simulink model "AC_base_1_VSM_2_22a"  (R2022a)
settings: Solver=ode3  StartTime=0.0  StopTime=8  FixedStep=HWSampleTime  RelTol=1e-3
undefined symbols (not defined in the file): ControlSampleTime, DiscIntNeverNeededParam, HWSampleTime, Ipwm_back, Ipwm_off, LCL, Manage, Oversample, Param, scaling_factor, SM, Ts, V_DC, VSMCTRL
libraries: fl_lib x100, nesl_utility x63, simulink x38, FriedrichLibrary x38, ee_lib x20, simulink_extras x14, TriphaseHardwaremodule x12, spsEdgeDetectorLib x2, StateMachines x2, slpidlib x2, spsPower3phInstantaneousLib x1
(part 6 of 7)

== system AC_base_1_VSM_2_22a/Variant Subsystem1/VSM/VSM1/VSM/MANAGEMENT/sp_VSM/PQ(U) Limit ==
  note: hier muss mit der Leistungsvorgabe multipliziert werden
      | 0.8 U * P0
  sp_PQ : Inport
  enable : Inport  Port=2
  u_out : Inport  Port=3
  Add : Sum
  Constant : Constant
  Dead Zone : DeadZone  LowerValue=0.95  UpperValue=1.05
  Demux : Demux  Outputs=2
  Demux1 : Demux  Outputs=2
  Math Function : Math  Operator=hypot  SignedPower=on
  MinMax : MinMax  Inputs=2
  Mux : Mux  Inputs=2
  Product : Product
  Scope : Scope
  Selector2 : Selector  InputPortWidth=3  IndexOptions=Index vector (dialog)  Indices=[1 2]  OutputSizes=1
  Switch : Switch  Criteria=u2 ~= 0  SaturateOnIntegerOverflow=off  InputSameDT=off
  sp_PQ_limit : Outport  VectorParamsAs1DForOutWhenUnconnected=off
  wires:
  Constant/1 -> Add/1
  Add/1 -> Product/1
  Dead Zone/1 -> Add/2
  Product/1 -> MinMax/1
  enable/1 -> Switch/2
  Switch/1 -> sp_PQ_limit/1, Scope/1
  Mux/1 -> Switch/1
  MinMax/1 -> Mux/1
  Demux1/1 -> Product/2, MinMax/2
  Demux1/2 -> Mux/2
  sp_PQ/1 -> Demux1/1, Switch/3
  u_out/1 -> Selector2/1
  Math Function/1 -> Dead Zone/1
  Demux/2 -> Math Function/2
  Demux/1 -> Math Function/1
  Selector2/1 -> Demux/1

== system AC_base_1_VSM_2_22a/Variant Subsystem1/VSM/VSM1/VSM/MANAGEMENT/sp_VSM/RateLimit ==
  PQ : Inport
  Enable : EnablePort
  Compare To Zero : simulink/Logic and Bit Operations/Compare To Zero  relop=>  OutDataTypeStr=boolean
  Constant1 : Constant  Value=Mgn.PQSpRateUp  SampleTime=ControlSampleTime
  Constant2 : Constant  Value=Mgn.PQSpRateDown  SampleTime=ControlSampleTime
  Constant6 : Constant  Value=Mgn.PQSpRateDown  SampleTime=ControlSampleTime
  Constant7 : Constant  Value=Mgn.PQSpRateUp  SampleTime=ControlSampleTime
  Constant8 : Constant  Value=[0 0]  SampleTime=ControlSampleTime
  Logical Operator : Logic  Inputs=1  AllPortsSameDT=off  OutDataTypeStr=boolean
  Mux : Mux  Inputs=2
  Switch : Switch  Criteria=u2 > Threshold  SaturateOnIntegerOverflow=off  InputSameDT=off
  ratelimitspPQ : Subsystem  mask{Ts=ControlSampleTime}
      mask DialogControl ParameterGroupVar Prompt: Rate Limiter
  PQslow : Outport  VectorParamsAs1DForOutWhenUnconnected=off
  wires:
  PQ/1 -> Switch/3, Switch/1, ratelimitspPQ/2(x)
  Constant8/1 -> ratelimitspPQ/4(x0)
  Constant6/1 -> ratelimitspPQ/3(ratedown)
  Switch/1 -> PQslow/1  "sp_PQ"
  Constant7/1 -> ratelimitspPQ/1(rateup)
  Compare To Zero/1 -> Logical Operator/1
  Constant1/1 -> Mux/1
  Constant2/1 -> Mux/2
  Mux/1 -> Compare To Zero/1
  Logical Operator/1 -> Switch/2

== system AC_base_1_VSM_2_22a/Variant Subsystem3/VSM/Inverter AverageMdl LC SimScape2/Modul F30 fixed DC voltage Average SimScape/simscape_bridgefilter_aca/PWM Blocking1/Trigger Spike at new Control Sample ==
  Add : Sum  Inputs=+-
  Compare To Constant : simulink/Logic and Bit Operations/Compare To Constant  relop=~=  const=0  OutDataTypeStr=boolean
  Rate Transition : RateTransition  OutPortSampleTime=ControlSampleTime
  Rate Transition1 : RateTransition  OutPortSampleTime=ControlSampleTime
  Rate Transition2 : RateTransition  OutPortSampleTime=ControlSampleTime/Oversample
  S-R Flip-Flop1 : simulink_extras/Flip Flops/S-R Flip-Flop  initial_condition=1
  Unit Delay : UnitDelay  SampleTime=-1  HasFrameUpgradeWarning=on
  Unit Delay2 : UnitDelay  SampleTime=-1  HasFrameUpgradeWarning=on
  Unit Delay3 : UnitDelay  SampleTime=-1  HasFrameUpgradeWarning=on
  y : Outport
  wires:
  S-R Flip-Flop1/1 -> Rate Transition2/1, Rate Transition/1
  Rate Transition2/1 -> Add/2, Unit Delay3/1
  S-R Flip-Flop1/2 -> Rate Transition1/1
  Unit Delay2/1 -> S-R Flip-Flop1/1
  Unit Delay3/1 -> Add/1
  Compare To Constant/1 -> y/1
  Add/1 -> Compare To Constant/1
  Unit Delay/1 -> S-R Flip-Flop1/2
  Rate Transition/1 -> Unit Delay/1
  Rate Transition1/1 -> Unit Delay2/1

== system AC_base_1_VSM_2_22a/Variant Subsystem3/VSM/Inverter AverageMdl LC SimScape2/Modul F30 fixed DC voltage Average SimScape/simscape_bridgefilter_aca1/PWM Blocking1/Trigger Spike at new Control Sample ==
  Add : Sum  Inputs=+-
  Compare To Constant : simulink/Logic and Bit Operations/Compare To Constant  relop=~=  const=0  OutDataTypeStr=boolean
  Rate Transition : RateTransition  OutPortSampleTime=ControlSampleTime
  Rate Transition1 : RateTransition  OutPortSampleTime=ControlSampleTime
  Rate Transition2 : RateTransition  OutPortSampleTime=ControlSampleTime/Oversample
  S-R Flip-Flop1 : simulink_extras/Flip Flops/S-R Flip-Flop  initial_condition=1
  Unit Delay : UnitDelay  SampleTime=-1  HasFrameUpgradeWarning=on
  Unit Delay2 : UnitDelay  SampleTime=-1  HasFrameUpgradeWarning=on
  Unit Delay3 : UnitDelay  SampleTime=-1  HasFrameUpgradeWarning=on
  y : Outport
  wires:
  Rate Transition1/1 -> Unit Delay2/1
  Rate Transition/1 -> Unit Delay/1
  Unit Delay/1 -> S-R Flip-Flop1/2
  Add/1 -> Compare To Constant/1
  Compare To Constant/1 -> y/1
  Unit Delay3/1 -> Add/1
  Unit Delay2/1 -> S-R Flip-Flop1/1
  S-R Flip-Flop1/2 -> Rate Transition1/1
  Rate Transition2/1 -> Unit Delay3/1, Add/2
  S-R Flip-Flop1/1 -> Rate Transition/1, Rate Transition2/1

== system AC_base_1_VSM_2_22a/Variant Subsystem3/VSM/Inverter AverageMdl LC SimScape2/Modul F30 fixed DC voltage Average SimScape/simscape_bridgefilter_aca2/PWM Blocking1/Trigger Spike at new Control Sample ==
  Add : Sum  Inputs=+-
  Compare To Constant : simulink/Logic and Bit Operations/Compare To Constant  relop=~=  const=0  OutDataTypeStr=boolean
  Rate Transition : RateTransition  OutPortSampleTime=ControlSampleTime
  Rate Transition1 : RateTransition  OutPortSampleTime=ControlSampleTime
  Rate Transition2 : RateTransition  OutPortSampleTime=ControlSampleTime/Oversample
  S-R Flip-Flop1 : simulink_extras/Flip Flops/S-R Flip-Flop  initial_condition=1
  Unit Delay : UnitDelay  SampleTime=-1  HasFrameUpgradeWarning=on
  Unit Delay2 : UnitDelay  SampleTime=-1  HasFrameUpgradeWarning=on
  Unit Delay3 : UnitDelay  SampleTime=-1  HasFrameUpgradeWarning=on
  y : Outport
  wires:
  S-R Flip-Flop1/1 -> Rate Transition2/1, Rate Transition/1
  Rate Transition2/1 -> Add/2, Unit Delay3/1
  S-R Flip-Flop1/2 -> Rate Transition1/1
  Unit Delay2/1 -> S-R Flip-Flop1/1
  Unit Delay3/1 -> Add/1
  Compare To Constant/1 -> y/1
  Add/1 -> Compare To Constant/1
  Unit Delay/1 -> S-R Flip-Flop1/2
  Rate Transition/1 -> Unit Delay/1
  Rate Transition1/1 -> Unit Delay2/1

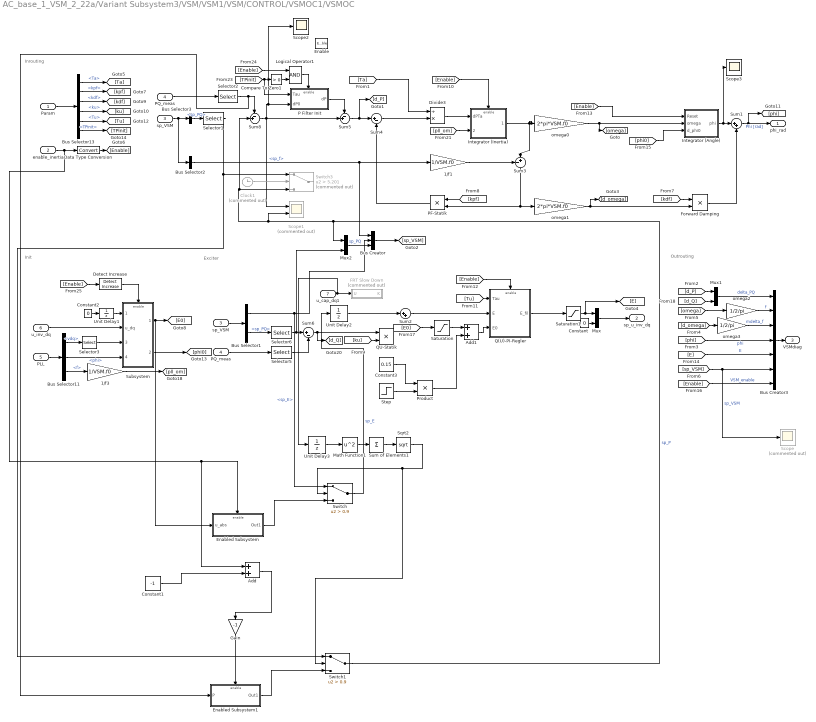
== system AC_base_1_VSM_2_22a/Variant Subsystem3/VSM/VSM1/VSM/CONTROL/VSMOC1/VSMOC ==
  note: Inrouting
  note: Exciter
  note: Init
  note: Outrouting
  Param : Inport
  enable_inertia : Inport  Port=2
  sp_VSM : Inport  Port=3
  PQ_meas : Inport  Port=4
  PLL : Inport  Port=5
  u_inv_dq : Inport  Port=6
  u_cap_dq1 : Inport  Port=7
  Enable : EnablePort  StatesWhenEnabling=reset
  1/f1 : Gain  Gain=1/VSM.f0
  1/f3 : Gain  Gain=1/VSM.f0
  Add : Sum
  Add1 : Sum
  Bus Creator : BusCreator  Inputs=3
  Bus Creator3 : BusCreator  Inputs=7
  Bus Selector1 : BusSelector  OutputSignals=sp_E,sp_PQ
  Bus Selector11 : BusSelector  OutputSignals=vdq,phi,f
  Bus Selector13 : BusSelector  OutputSignals=Ta,kpf,kdf,ku,Tu,TPinit
  Bus Selector2 : BusSelector  OutputSignals=sp_f
  Bus Selector3 : BusSelector  OutputSignals=sp_PQ
  Clock1 : Clock  Commented=on
  Compare To Zero1 : simulink/Logic and Bit Operations/Compare To Zero  relop=>  OutDataTypeStr=boolean
  Constant : Constant  Value=0
  Constant1 : Constant  Value=-1
  Constant2 : Constant  Value=0  SampleTime=ControlSampleTime
  Constant3 : Constant  Value=0.15
  Data Type Conversion : DataTypeConversion  SaturateOnIntegerOverflow=off  RndMeth=Floor
  Detect Increase : simulink/Logic and Bit Operations/Detect Increase  vinit=0.0  OutDataTypeStr=boolean
  Divide3 : Product  Inputs=/*
  Enabled Subsystem : Subsystem  TreatAsAtomicUnit=on
  Enabled Subsystem1 : Subsystem  TreatAsAtomicUnit=on
  FRT Slow Down : Subsystem  Commented=on
  Forward Damping : Product  Inputs=**
  Gain : Gain  Gain=-1
  Integrator (Angle) : Subsystem
  Integrator (Inertia) : Subsystem
  Logical Operator1 : Logic  AllPortsSameDT=off  OutDataTypeStr=boolean
  Math Function1 : Math  Operator=square  SignedPower=on
  Mux : Mux  Inputs=2
  Mux1 : Mux  Inputs=2
  Mux2 : Mux  Inputs=2
  P Filter Init : Subsystem
  PF-Statik : Product  Inputs=**
  "PQ_meas " : InportShadow  Port=4
  Product : Product
  Q(U)-PI-Regler : Subsystem
  QU-Statik : Product  Inputs=**
  Saturation : Saturate  UpperLimit=1.8  LowerLimit=0.8*0
  Saturation1 : Saturate  UpperLimit=2
  Scope : Scope  Commented=on
  Scope1 : Scope  Commented=on  NumInputPorts=2
  Scope2 : Scope
  Scope3 : Scope
  Selector1 : Selector  InputPortWidth=2  IndexOptions=Index vector (dialog)  Indices=1  OutputSizes=1
  Selector2 : Selector  InputPortWidth=2  IndexOptions=Index vector (dialog)  Indices=1  OutputSizes=1
  Selector3 : Selector  InputPortWidth=3  IndexOptions=Index vector (dialog)  Indices=[1 2]  OutputSizes=1
  Selector5 : Selector  InputPortWidth=2  IndexOptions=Index vector (dialog)  Indices=2  OutputSizes=1
  Selector6 : Selector  InputPortWidth=2  IndexOptions=Index vector (dialog)  Indices=2  OutputSizes=1
  Sqrt2 : Sqrt
  Step : Step  Time=2  After=0  SampleTime=0
  Subsystem : Subsystem
  Sum of Elements1 : Sum  Inputs=+
  Sum1 : Sum  Inputs=|++
  Sum2 : Sum  Inputs=|++
  Sum3 : Sum  Inputs=-+|
  Sum4 : Sum  Inputs=|+-
  Sum5 : Sum  Inputs=-+|
  Sum6 : Sum  Inputs=|+-
  Sum8 : Sum  Inputs=-+|
  Switch : Switch  Criteria=u2 > Threshold  Threshold=0.9  SaturateOnIntegerOverflow=off  InputSameDT=off
  Switch1 : Switch  Criteria=u2 > Threshold  Threshold=0.9  SaturateOnIntegerOverflow=off  InputSameDT=off
  Switch3 : Switch  Commented=on  Criteria=u2 > Threshold  Threshold=5.201  SaturateOnIntegerOverflow=off  InputSameDT=off
  Unit Delay1 : UnitDelay  InitialCondition=1  SampleTime=ControlSampleTime  HasFrameUpgradeWarning=on
  Unit Delay2 : UnitDelay  SampleTime=-1  HasFrameUpgradeWarning=on
  Unit Delay3 : UnitDelay  SampleTime=-1  HasFrameUpgradeWarning=on
  omega0 : Gain  Gain=2*pi*VSM.f0
  omega1 : Gain  Gain=2*pi*VSM.f0
  omega2 : Gain  Gain=1/2/pi
  omega3 : Gain  Gain=1/2/pi
  "sp_VSM " : InportShadow  Port=3
  phi_rad : Outport  VectorParamsAs1DForOutWhenUnconnected=off
  sp_u_inv_dq : Outport  Port=2  InitialOutput=[1 0]  VectorParamsAs1DForOutWhenUnconnected=off
  VSMdiag : Outport  Port=3  VectorParamsAs1DForOutWhenUnconnected=off
  wires:
  [Enable] -> Q(U)-PI-Regler/Enable
  Bus Selector11/2 -> Subsystem/4(phi_pll)  "<phi>"
  Selector5/1 -> Sum6/2
  Selector6/1 -> Mux2/2, Sum6/1
  1/f1/1 -> Sum3/1
  [d_Q] -> Mux1/2
  [d_P] -> Mux1/1
  Mux1/1 -> Bus Creator3/1  "delta_PQ"
  Selector2/1 -> Enabled Subsystem1/1(P), Sum8/1
  Sum6/1 -> QU-Statik/1, [d_Q]
  "sp_VSM "/1 -> Bus Selector1/1
  Bus Selector1/2 -> Selector6/1  "<sp_PQ>"
  "PQ_meas "/1 -> Selector5/1
  [kpf] -> PF-Statik/1
  [kdf] -> Forward Damping/1
  1/f3/1 -> [pll_om]
  Bus Selector11/3 -> 1/f3/1  "<f>"
  Integrator (Angle)/1(phi) -> Scope3/1, Sum1/1
  Selector3/1 -> Subsystem/3(u_dq_pll)
  [Enable] -> Bus Creator3/7  "VSM_enable"
  Sum1/1 -> [phi], phi_rad/1  "Phi [rad]"
  Sum4/1 -> Divide3/2
  Sum3/1 -> PF-Statik/2, omega1/1
  Bus Selector2/1 -> Bus Creator/1, 1/f1/1  "<sp_f>"
  PLL/1 -> Bus Selector11/1
  Bus Creator3/1 -> VSMdiag/1
  [omega] -> omega2/1
  omega1/1 -> Forward Damping/2, [d_omega]
  [d_omega] -> omega3/1
  omega2/1 -> Bus Creator3/2  "f"
  omega3/1 -> Bus Creator3/3  "mdelta_f"
  [sp_VSM] -> Scope/1, Bus Creator3/6  "sp_VSM"
  PQ_meas/1 -> Selector2/1
  Bus Selector11/1 -> Selector3/1  "<vdq>"
  Divide3/1 -> Integrator (Inertia)/1(dPTa)
  [pll_om] -> Integrator (Inertia)/2(omega0 [pu])
  Mux/1 -> sp_u_inv_dq/1
  Constant/1 -> Mux/2
  Subsystem/2(u_ang) -> [phi0]
  Detect Increase/1 -> Subsystem/Enable
  Sum5/1 -> Sum4/1, [d_P]
  [TPinit] -> P Filter Init/1(Tau), Compare To Zero1/1
  Compare To Zero1/1 -> Logical Operator1/2
  Logical Operator1/1 -> P Filter Init/Enable
  [Enable] -> Logical Operator1/1
  Bus Selector13/5 -> [Tu]  "<Tu>"
  Bus Selector13/4 -> [ku]  "<ku>"
  Bus Selector13/3 -> [kdf]  "<kdf>"
  Bus Selector13/2 -> [kpf]  "<kpf>"
  Bus Selector13/1 -> [Ta]  "<Ta>"
  Param/1 -> Bus Selector13/1
  [Enable] -> Detect Increase/1
  u_inv_dq/1 -> Subsystem/2(u_dq)
  Constant2/1 -> Unit Delay1/1
  Unit Delay1/1 -> Subsystem/1(first_run)
  Data Type Conversion/1 -> [Enable]
  Sum2/1 -> Q(U)-PI-Regler/2(E)
  [ku] -> QU-Statik/2
  [E] -> Bus Creator3/5  "E"
  Bus Selector13/6 -> [TPinit]  "<TPinit>"
  [phi] -> Bus Creator3/4  "phi"
  [Tu] -> Q(U)-PI-Regler/1(Tau)
  Unit Delay2/1 -> Sum2/1
  [E0] -> Saturation/1
  [Enable] -> Integrator (Angle)/1(Reset)
  omega0/1 -> Integrator (Angle)/2(omega), [omega]
  Saturation1/1 -> [E], Mux/1
  Forward Damping/1 -> Sum1/2
  [Enable] -> Integrator (Inertia)/Enable
  Integrator (Inertia)/1(omega [pu]) -> omega0/1, Sum3/2
  Bus Selector3/1 -> Selector1/1  "<sp_PQ>"
  sp_VSM/1 -> Bus Selector2/1, Bus Selector3/1
  Sum8/1 -> Scope1/1, Sum5/2, Scope2/1, P Filter Init/2(dP0)
  [phi0] -> Integrator (Angle)/3(d_phi0)
  [Ta] -> Divide3/1
  P Filter Init/1(dP) -> Sum5/1
  PF-Statik/1 -> Sum4/2
  Sqrt2/1 -> Switch1/2, Switch/2
  u_cap_dq1/1 -> Unit Delay3/1, FRT Slow Down/1(U)
  Sum of Elements1/1 -> Sqrt2/1
  Unit Delay3/1 -> Math Function1/1
  Math Function1/1 -> Sum of Elements1/1
  Bus Selector1/1 -> Bus Creator/2, Switch/1  "<sp_E>"
  enable_inertia/1 -> Add/1, Enabled Subsystem/Enable, Data Type Conversion/1
  Enabled Subsystem/1(Out1) -> Switch/3
  Subsystem/1(u_abs) -> Enabled Subsystem/1(u_abs), [E0]
  Enabled Subsystem1/1(Out1) -> Switch1/3
  Switch/1 -> Unit Delay2/1  "sp_E"
  Switch1/1 -> Scope1/2, Sum8/2, Switch3/3, Mux2/1  "sp_P"
  Clock1/1 -> Switch3/2
  Q(U)-PI-Regler/1(E_fil) -> Saturation1/1
  Selector1/1 -> Switch3/1, Switch1/1
  Constant1/1 -> Add/2
  Gain/1 -> Enabled Subsystem1/Enable
  Add/1 -> Gain/1
  Saturation/1 -> Add1/1
  Add1/1 -> Q(U)-PI-Regler/3(E0)
  Step/1 -> Product/2
  Constant3/1 -> Product/1
  Product/1 -> Add1/2
  Mux2/1 -> Bus Creator/3  "sp_PQ"
  Bus Creator/1 -> [sp_VSM]

== system AC_base_1_VSM_2_22a/Variant Subsystem3/VSM/VSM1/VSM/CONTROL/Virtual Circuit mit R und L/Current Predictor ==
  u : Inport
  Delay : Delay  DelayLength=1  InitialCondition=0
  Sum : Sum  Inputs=|-+
  Sum1 : Sum  Inputs=|++
  y : Outport
  wires:
  u/1 -> Sum/2, Sum1/2, Delay/1
  Delay/1 -> Sum/1
  Sum/1 -> Sum1/1
  Sum1/1 -> y/1

== system AC_base_1_VSM_2_22a/Variant Subsystem3/VSM/VSM1/VSM/CONTROL/Virtual Circuit mit R und L/PT1 ==
  U : Inport  SampleTime=Ts
  tau : Inport  Port=2  SampleTime=Ts
  Reset : Inport  Port=3  SampleTime=Ts
  Phi : Inport  Port=4
  Delay : Delay  DelayLength=1  InitialConditionSource=Input port  ExternalReset=Rising
      settings: InputPortMap=u0,r5,p4
  Divide : Product  Inputs=*/
  Gain : Gain  Gain=Ts
  Gain1 : Gain  Gain=K
  Saturation : Saturate  UpperLimit=inf  LowerLimit=Ts
  Sum : Sum  Inputs=|++
  Sum2 : Sum  Inputs=|+-
  Unit Delay2 : UnitDelay  InitialCondition=[0 0 0]  SampleTime=ControlSampleTime  HasFrameUpgradeWarning=on
  dq0->ab0 phi : FriedrichLibrary/Transformations/dq0->ab0 phi  SystemSampleTime=-1  VariantActivationTime=update diagram  Latency=0  AutoFrameSizeCalculation=off
  Y : Outport
  wires:
  Phi/1 -> dq0->ab0 phi/2
  Unit Delay2/1 -> dq0->ab0 phi/1
  Sum/1 -> Gain1/1, Unit Delay2/1, Delay/1
  Reset/1 -> Delay/2
  Saturation/1 -> Divide/2
  Divide/1 -> Sum/1
  tau/1 -> Saturation/1
  Delay/1 -> Sum2/2, Sum/2
  Gain/1 -> Divide/1
  U/1 -> Sum2/1
  Sum2/1 -> Gain/1
  Gain1/1 -> Y/1
  dq0->ab0 phi/1 -> Delay/3

== system AC_base_1_VSM_2_22a/Variant Subsystem3/VSM/VSM1/VSM/CONTROL/Virtual Circuit mit R und L/PT2 ==
  U : Inport  SampleTime=Ts
  tau : Inport  Port=2  SampleTime=Ts
  Reset : Inport  Port=3  SampleTime=Ts
  Phi : Inport  Port=4
  Delay : Delay  DelayLength=1  InitialConditionSource=Input port  ExternalReset=Rising
      settings: InputPortMap=u0,r5,p4
  Divide : Product  Inputs=*/
  Gain : Gain  Gain=Ts
  Gain1 : Gain  Gain=K
  Saturation : Saturate  UpperLimit=inf  LowerLimit=Ts
  Sum : Sum  Inputs=|++
  Sum2 : Sum  Inputs=|+-
  Unit Delay2 : UnitDelay  InitialCondition=[0 0 0]  SampleTime=ControlSampleTime  HasFrameUpgradeWarning=on
  dq0->ab0 phi1 : FriedrichLibrary/Transformations/dq0->ab0 phi  SystemSampleTime=-1  VariantActivationTime=update diagram  Latency=0  AutoFrameSizeCalculation=off
  Y : Outport
  wires:
  dq0->ab0 phi1/1 -> Delay/3
  Gain1/1 -> Y/1
  Sum2/1 -> Gain/1
  U/1 -> Sum2/1
  Gain/1 -> Divide/1
  Delay/1 -> Sum/2, Sum2/2
  tau/1 -> Saturation/1
  Divide/1 -> Sum/1
  Saturation/1 -> Divide/2
  Reset/1 -> Delay/2
  Sum/1 -> Delay/1, Unit Delay2/1, Gain1/1
  Unit Delay2/1 -> dq0->ab0 phi1/1
  Phi/1 -> dq0->ab0 phi1/2

== system AC_base_1_VSM_2_22a/Variant Subsystem3/VSM/VSM1/VSM/CONTROL/Virtual Circuit1/Current Predictor ==
  u : Inport
  Delay : Delay  DelayLength=1  InitialCondition=0
  Sum : Sum  Inputs=|-+
  Sum1 : Sum  Inputs=|++
  y : Outport
  wires:
  u/1 -> Sum/2, Sum1/2, Delay/1
  Delay/1 -> Sum/1
  Sum/1 -> Sum1/1
  Sum1/1 -> y/1

== system AC_base_1_VSM_2_22a/Variant Subsystem3/VSM/VSM1/VSM/CONTROL/Virtual Circuit1/PT1 ==
  U : Inport  SampleTime=Ts
  tau : Inport  Port=2  SampleTime=Ts
  Reset : Inport  Port=3  SampleTime=Ts
  Delay : Delay  DelayLength=1
  Divide : Product  Inputs=*/
  Gain : Gain  Gain=Ts
  Gain1 : Gain  Gain=K
  Saturation : Saturate  UpperLimit=inf  LowerLimit=Ts
  Sum : Sum  Inputs=|++
  Sum2 : Sum  Inputs=|+-
  Switch : Switch  Criteria=u2 > Threshold  SaturateOnIntegerOverflow=off  InputSameDT=off
  Y : Outport
  wires:
  Reset/1 -> Switch/2
  Saturation/1 -> Divide/2
  Divide/1 -> Sum/1
  tau/1 -> Saturation/1
  Delay/1 -> Sum2/2, Sum/2
  Gain/1 -> Divide/1
  U/1 -> Switch/1, Sum2/1
  Sum2/1 -> Gain/1
  Gain1/1 -> Y/1
  Switch/1 -> Gain1/1, Delay/1
  Sum/1 -> Switch/3

== system AC_base_1_VSM_2_22a/Variant Subsystem3/VSM/VSM1/VSM/CONTROL/Virtual Circuit1/PT2 ==
  U : Inport  SampleTime=Ts
  tau : Inport  Port=2  SampleTime=Ts
  Reset : Inport  Port=3  SampleTime=Ts
  Phi : Inport  Port=4
  Delay : Delay  DelayLength=1  InitialConditionSource=Input port  ExternalReset=Rising
      settings: InputPortMap=u0,r5,p4
  Divide : Product  Inputs=*/
  Gain : Gain  Gain=Ts
  Gain1 : Gain  Gain=K
  Saturation : Saturate  UpperLimit=inf  LowerLimit=Ts
  Sum : Sum  Inputs=|++
  Sum2 : Sum  Inputs=|+-
  Unit Delay2 : UnitDelay  InitialCondition=[0 0 0]  SampleTime=ControlSampleTime  HasFrameUpgradeWarning=on
  dq0->ab0 phi1 : FriedrichLibrary/Transformations/dq0->ab0 phi  SystemSampleTime=-1  VariantActivationTime=update diagram  Latency=0  AutoFrameSizeCalculation=off
  Y : Outport
  wires:
  dq0->ab0 phi1/1 -> Delay/3
  Gain1/1 -> Y/1
  Sum2/1 -> Gain/1
  U/1 -> Sum2/1
  Gain/1 -> Divide/1
  Delay/1 -> Sum/2, Sum2/2
  tau/1 -> Saturation/1
  Divide/1 -> Sum/1
  Saturation/1 -> Divide/2
  Reset/1 -> Delay/2
  Sum/1 -> Delay/1, Unit Delay2/1, Gain1/1
  Unit Delay2/1 -> dq0->ab0 phi1/1
  Phi/1 -> dq0->ab0 phi1/2

== system AC_base_1_VSM_2_22a/Variant Subsystem3/VSM/VSM1/VSM/CONTROL/i_dq_ctrl/PI ==
  di : Inport
  u0 : Inport  Port=2
  Enable : EnablePort  StatesWhenEnabling=reset
  Gain4 : Gain  Gain=Ki
  Gain5 : Gain  Gain=Kp
  Integrator (inertia) : DiscreteIntegrator  gainval=1  InitialConditionSource=external  InitialCondition=1  SampleTime=ControlSampleTime  ICPrevOutput=DiscIntNeverNeededParam  ICPrevScaledInput=DiscIntNeverNeededParam
  Product : Product
  Product1 : Product
  Step : Step  Time=8  Before=1  SampleTime=0
  Step1 : Step  Time=8.05+10  Before=1  After=0.1  SampleTime=0
  Sum2 : Sum  Inputs=++|
  u : Outport  VectorParamsAs1DForOutWhenUnconnected=off
  wires:
  u0/1 -> Integrator (inertia)/2
  Sum2/1 -> u/1
  di/1 -> Gain4/1, Gain5/1
  Integrator (inertia)/1 -> Sum2/2
  Gain5/1 -> Product/2
  Gain4/1 -> Product1/2
  Product1/1 -> Integrator (inertia)/1
  Product/1 -> Sum2/1
  Step/1 -> Product/1
  Step1/1 -> Product1/1

== system AC_base_1_VSM_2_22a/Variant Subsystem3/VSM/VSM1/VSM/MANAGEMENT/Subsystem1/Enabled Subsystem ==
  i_abs : Inport
  i_pq : Inport  Port=2
  Enable : EnablePort
  i abs_pre : Outport
  i_pq_pre : Outport  Port=2
  wires:
  i_abs/1 -> i abs_pre/1
  i_pq/1 -> i_pq_pre/1

== system AC_base_1_VSM_2_22a/Variant Subsystem3/VSM/VSM1/VSM/MANAGEMENT/Subsystem1/Subsystem ==
  note: für mean muss simscape installiert sein
  note: zweiter Faktor bei clearing für richtiges Q
      |
      | bei Eintritt mit Halten aber fester Grenze
      |
      | bis jetzt über Zeit abgeschaltet bei clearing ohne Halten
  i_inv : Inport
  PQ_out : Inport  Port=2
  iabs : Inport  Port=3
  U_cap : Inport  Port=4
  PQ_pre : Inport  Port=5
  i abs_pre : Inport  Port=6
  angle_i : Inport  Port=7
  Enable : EnablePort
  Abs : Abs  SaturateOnIntegerOverflow=off
  Add : Sum  Inputs=+-
  Clock : Clock
  Complex to Magnitude-Angle : ComplexToMagnitudeAngle
  Demux1 : Demux  Outputs=2
  Discrete Derivative2 : simulink/Discrete/Discrete Derivative  gainval=1.0  ICPrevScaledInput=0.0  OutMin=[]  OutMax=[]  OutDataType=fixdt(1, 16)  OutScaling=2^-10  DoSatur=off
  Discrete-Time Integrator : DiscreteIntegrator  SampleTime=-1  ICPrevOutput=DiscIntNeverNeededParam  ICPrevScaledInput=DiscIntNeverNeededParam
  Divide2 : Product  Inputs=*/
  Gain : Gain  Gain=1000  SaturateOnIntegerOverflow=on  OutDataTypeStr=Inherit: Same as input  ParamDataTypeStr=Inherit: Same as input
  K1 : Constant  Value=1./1000  SampleTime=Ts
  MATLAB Function1 : MATLAB Function  TreatAsAtomicUnit=on  SystemSampleTime=ControlSampleTime
  MATLAB Function2 : MATLAB Function  Commented=on  TreatAsAtomicUnit=on  SystemSampleTime=ControlSampleTime
  Memory : Memory
  Real-Imag to Complex : RealImagToComplex
  Relational Operator : RelationalOperator  OutDataTypeStr=boolean  ZeroCross=off  SampleTime=Ts  InputSameDT=off
  Scope1 : Scope  NumInputPorts=2
  Scope2 : Scope  NumInputPorts=2
  Selector3 : Selector  InputPortWidth=2  IndexOptions=Index vector (dialog)  Indices=2  OutputSizes=1
  Signal Specification9 : SignalSpecification  Dimensions=[1 2]
  Sum : Sum  Inputs=+-  InputSameDT=on  SaturateOnIntegerOverflow=on  OutDataTypeStr=Inherit: Same as first input
  Switch : Switch  Threshold=0.5  SaturateOnIntegerOverflow=off
  Transport Delay : TransportDelay  DelayTime=0.002
  Transport Delay1 : TransportDelay  DelayTime=1./1000  BufferSize=2048*4  PadeOrder=2
  i_sp : Outport
  CC : Outport  Port=2
  set : Outport  Port=3
  wires:
  PQ_out/1 -> MATLAB Function1/2(PQ_out), Divide2/1
  iabs/1 -> MATLAB Function1/3(i_abs)
  U_cap/1 -> MATLAB Function1/5(U_cap), Divide2/2, Add/1, Transport Delay/1
  MATLAB Function1/1(i_sp) -> Signal Specification9/1
  MATLAB Function1/2(CC) -> CC/1
  i abs_pre/1 -> MATLAB Function1/7(i_abs_pre)
  Transport Delay/1 -> Add/2
  Add/1 -> MATLAB Function1/8(u_diff)
  i_inv/1 -> MATLAB Function1/1(i_inv)
  Discrete Derivative2/1 -> Abs/1
  MATLAB Function1/3(set1) -> set/1, Scope1/1
  Divide2/1 -> Selector3/1, Scope2/1
  Selector3/1 -> Discrete Derivative2/1
  Demux1/1 -> Real-Imag to Complex/1
  PQ_pre/1 -> MATLAB Function1/6(i_pq_pre), Demux1/1
  Complex to Magnitude-Angle/2 -> MATLAB Function1/9(angle_pre)
  Demux1/2 -> Real-Imag to Complex/2
  Real-Imag to Complex/1 -> Complex to Magnitude-Angle/1
  angle_i/1 -> MATLAB Function1/10(angle_i)
  Signal Specification9/1 -> i_sp/1
  Relational Operator/1 -> Switch/2
  Memory/1 -> Switch/3
  Discrete-Time Integrator/1 -> Sum/1, Transport Delay1/1
  Sum/1 -> Gain/1
  Gain/1 -> Switch/1
  Clock/1 -> Relational Operator/1
  K1/1 -> Relational Operator/2
  Transport Delay1/1 -> Sum/2
  Abs/1 -> Discrete-Time Integrator/1
  Switch/1 -> MATLAB Function1/4(der), Scope2/2, Memory/1

== system AC_base_1_VSM_2_22a/Variant Subsystem3/VSM/VSM1/VSM/MANAGEMENT/sp_VSM/E(PQ) ==
  E : Inport
  cmd : Inport  Port=2
  sp_PQ : Inport  Port=3
  Abs : Abs  SaturateOnIntegerOverflow=off
  Add : Sum
  Add1 : Sum  Inputs=--
  Add2 : Sum  Inputs=+++
  Bus Selector : BusSelector  OutputSignals=Param.VC.R1,Param.VC.R1t,Param.VC.L1,Param.VC.L1t,Param.VSM.ku
  Bus Selector1 : BusSelector  OutputSignals=Param.VSM.sp_E_comp
  Constant : Constant
  Demux : Demux  Outputs=2
  Display{,1..4} (5 alike) : Display
  Divide : Product  Inputs=/*
  Product : Product
  Product1 : Product
  Real-Imag to Complex : RealImagToComplex
  Real-Imag to Complex1 : RealImagToComplex
  Switch : Switch  Criteria=u2 ~= 0  SaturateOnIntegerOverflow=off  InputSameDT=off
  "cmd " : InportShadow  Port=2
  sp_E : Outport  VectorParamsAs1DForOutWhenUnconnected=off
  wires:
  Add2/1 -> Display3/1, Abs/1
  Abs/1 -> Display4/1, Switch/1
  Product/1 -> Display2/1, Add2/2  "voltage"
  Real-Imag to Complex/1 -> Display1/1, Product/2  "impedance"
  Divide/1 -> Display/1, Product/1  "current"
  Real-Imag to Complex1/1 -> Divide/2
  Demux/2 -> Product1/1, Real-Imag to Complex1/2
  Demux/1 -> Real-Imag to Complex1/1
  sp_PQ/1 -> Demux/1
  E/1 -> Switch/3
  Add1/1 -> Real-Imag to Complex/2
  Add/1 -> Real-Imag to Complex/1
  Bus Selector/4 -> Add1/2  "<L1t>"
  Bus Selector/3 -> Add1/1  "<L1>"
  Bus Selector/2 -> Add/2  "<R1t>"
  Bus Selector/1 -> Add/1  "<R1>"
  cmd/1 -> Bus Selector/1
  Switch/1 -> sp_E/1
  "cmd "/1 -> Bus Selector1/1
  Bus Selector1/1 -> Switch/2  "<sp_E_comp>"
  Bus Selector/5 -> Product1/2  "<ku>"
  Product1/1 -> Add2/3
  Constant/1 -> Divide/1, Add2/1

== system AC_base_1_VSM_2_22a/Variant Subsystem3/VSM/VSM1/VSM/MANAGEMENT/sp_VSM/PQ(U) Limit ==
  note: hier muss mit der Leistungsvorgabe multipliziert werden
      | 0.8 U * P0
  sp_PQ : Inport
  enable : Inport  Port=2
  u_out : Inport  Port=3
  Add : Sum
  Constant : Constant
  Dead Zone : DeadZone  LowerValue=0.95  UpperValue=1.05
  Demux : Demux  Outputs=2
  Demux1 : Demux  Outputs=2
  Math Function : Math  Operator=hypot  SignedPower=on
  MinMax : MinMax  Inputs=2
  Mux : Mux  Inputs=2
  Product : Product
  Scope : Scope
  Selector2 : Selector  InputPortWidth=3  IndexOptions=Index vector (dialog)  Indices=[1 2]  OutputSizes=1
  Switch : Switch  Criteria=u2 ~= 0  SaturateOnIntegerOverflow=off  InputSameDT=off
  sp_PQ_limit : Outport  VectorParamsAs1DForOutWhenUnconnected=off
  wires:
  Selector2/1 -> Demux/1
  Demux/1 -> Math Function/1
  Demux/2 -> Math Function/2
  Math Function/1 -> Dead Zone/1
  u_out/1 -> Selector2/1
  sp_PQ/1 -> Switch/3, Demux1/1
  Demux1/2 -> Mux/2
  Demux1/1 -> MinMax/2, Product/2
  MinMax/1 -> Mux/1
  Mux/1 -> Switch/1
  Switch/1 -> Scope/1, sp_PQ_limit/1
  enable/1 -> Switch/2
  Product/1 -> MinMax/1
  Dead Zone/1 -> Add/2
  Add/1 -> Product/1
  Constant/1 -> Add/1

== system AC_base_1_VSM_2_22a/Variant Subsystem3/VSM/VSM1/VSM/MANAGEMENT/sp_VSM/RateLimit ==
  PQ : Inport
  Enable : EnablePort
  Compare To Zero : simulink/Logic and Bit Operations/Compare To Zero  relop=>  OutDataTypeStr=boolean
  Constant1 : Constant  Value=Mgn.PQSpRateUp  SampleTime=ControlSampleTime
  Constant2 : Constant  Value=Mgn.PQSpRateDown  SampleTime=ControlSampleTime
  Constant6 : Constant  Value=Mgn.PQSpRateDown  SampleTime=ControlSampleTime
  Constant7 : Constant  Value=Mgn.PQSpRateUp  SampleTime=ControlSampleTime
  Constant8 : Constant  Value=[0 0]  SampleTime=ControlSampleTime
  Logical Operator : Logic  Inputs=1  AllPortsSameDT=off  OutDataTypeStr=boolean
  Mux : Mux  Inputs=2
  Switch : Switch  Criteria=u2 > Threshold  SaturateOnIntegerOverflow=off  InputSameDT=off
  ratelimitspPQ : Subsystem  mask{Ts=ControlSampleTime}
      mask DialogControl ParameterGroupVar Prompt: Rate Limiter
  PQslow : Outport  VectorParamsAs1DForOutWhenUnconnected=off
  wires:
  Logical Operator/1 -> Switch/2
  Mux/1 -> Compare To Zero/1
  Constant2/1 -> Mux/2
  Constant1/1 -> Mux/1
  Compare To Zero/1 -> Logical Operator/1
  Constant7/1 -> ratelimitspPQ/1(rateup)
  Switch/1 -> PQslow/1  "sp_PQ"
  Constant6/1 -> ratelimitspPQ/3(ratedown)
  Constant8/1 -> ratelimitspPQ/4(x0)
  PQ/1 -> ratelimitspPQ/2(x), Switch/1, Switch/3

== system AC_base_1_VSM_2_22a/Variant Subsystem1/VSM/VSM1/VSM/CONTROL/VSMOC1/VSMOC/Enabled Subsystem ==
  u_abs : Inport
  Enable : EnablePort
  Out1 : Outport
  wires:
  u_abs/1 -> Out1/1

== system AC_base_1_VSM_2_22a/Variant Subsystem1/VSM/VSM1/VSM/CONTROL/VSMOC1/VSMOC/Enabled Subsystem1 ==
  P : Inport
  Enable : EnablePort
  Out1 : Outport
  wires:
  P/1 -> Out1/1

== system AC_base_1_VSM_2_22a/Variant Subsystem1/VSM/VSM1/VSM/CONTROL/VSMOC1/VSMOC/FRT Slow Down ==
  U : Inport
  Bias : Bias  Bias=0.2  SaturateOnIntegerOverflow=off
  Complex to Magnitude-Angle : ComplexToMagnitudeAngle
  Demux : Demux  Outputs=2
  Real-Imag to Complex : RealImagToComplex
  Saturation : Saturate  UpperLimit=1  LowerLimit=0
  Terminator : Terminator
  Unit Delay4 : UnitDelay  SampleTime=ControlSampleTime  HasFrameUpgradeWarning=on
  K : Outport  VectorParamsAs1DForOutWhenUnconnected=off
  wires:
  Unit Delay4/1 -> Demux/1
  Saturation/1 -> K/1
  Bias/1 -> Saturation/1
  Complex to Magnitude-Angle/2 -> Terminator/1
  U/1 -> Unit Delay4/1
  Real-Imag to Complex/1 -> Complex to Magnitude-Angle/1
  Demux/1 -> Real-Imag to Complex/1
  Demux/2 -> Real-Imag to Complex/2
  Complex to Magnitude-Angle/1 -> Bias/1

== system AC_base_1_VSM_2_22a/Variant Subsystem1/VSM/VSM1/VSM/CONTROL/VSMOC1/VSMOC/Integrator (Angle) ==
  Reset : Inport
  omega : Inport  Port=2
  d_phi0 : Inport  Port=3
  Angle Integrator Reset[SI] : FriedrichLibrary/Discrete Stuff/Angle Integrator Reset[SI]  Ts=ControlSampleTime
  Delay : Delay  DelayLength=1  InitialConditionSource=Input port
      settings: InputPortMap=u0,p4
  Gain3 : Gain  Gain=-1*ControlSampleTime
  Scope : Scope  NumInputPorts=2
  Scope1 : Scope  NumInputPorts=2
  Sum1 : Sum  Inputs=|++
  Sum9 : Sum  Inputs=|+-
  phi : Outport  VectorParamsAs1DForOutWhenUnconnected=off
  wires:
  Delay/1 -> Sum1/2, Scope/1
  d_phi0/1 -> Sum9/1
  Sum1/1 -> Angle Integrator Reset[SI]/3, Scope1/2
  Sum9/1 -> Sum1/1
  Reset/1 -> Angle Integrator Reset[SI]/1, Scope1/1
  Angle Integrator Reset[SI]/1 -> phi/1, Delay/1  "Phi [rad]"
  omega/1 -> Angle Integrator Reset[SI]/2, Gain3/1
  Gain3/1 -> Delay/2, Scope/2, Sum9/2

== system AC_base_1_VSM_2_22a/Variant Subsystem1/VSM/VSM1/VSM/CONTROL/VSMOC1/VSMOC/Integrator (Inertia) ==
  dPTa : Inport
  omega0 [pu] : Inport  Port=2
  Enable : EnablePort
  Integrator (inertia) : DiscreteIntegrator  gainval=1  InitialConditionSource=external  InitialCondition=1  SampleTime=ControlSampleTime  ICPrevOutput=DiscIntNeverNeededParam  ICPrevScaledInput=DiscIntNeverNeededParam
  omega [pu] : Outport  VectorParamsAs1DForOutWhenUnconnected=off
  wires:
  dPTa/1 -> Integrator (inertia)/1
  Integrator (inertia)/1 -> omega [pu]/1  "Omega [pu]"
  omega0 [pu]/1 -> Integrator (inertia)/2

== system AC_base_1_VSM_2_22a/Variant Subsystem1/VSM/VSM1/VSM/CONTROL/VSMOC1/VSMOC/P Filter Init ==
  Tau : Inport
  dP0 : Inport  Port=2
  Enable : EnablePort  StatesWhenEnabling=reset
  Divide4 : Product  Inputs=*/
  Gain : Gain  Gain=-1
  Integrator1 : DiscreteIntegrator  gainval=1  InitialConditionSource=external  SampleTime=ControlSampleTime  ICPrevOutput=DiscIntNeverNeededParam  ICPrevScaledInput=DiscIntNeverNeededParam
  dP : Outport  VectorParamsAs1DForOutWhenUnconnected=off
  wires:
  Integrator1/1 -> Gain/1, dP/1
  Tau/1 -> Divide4/2
  Divide4/1 -> Integrator1/1
  Gain/1 -> Divide4/1
  dP0/1 -> Integrator1/2

== system AC_base_1_VSM_2_22a/Variant Subsystem1/VSM/VSM1/VSM/CONTROL/VSMOC1/VSMOC/Q(U)-PI-Regler ==
  Tau : Inport
  E : Inport  Port=2
  E0 : Inport  Port=3
  Enable : EnablePort  StatesWhenEnabling=reset
  Divide2 : Product  Inputs=*/
  Integrator : DiscreteIntegrator  gainval=1  InitialConditionSource=external  InitialCondition=0.9  SampleTime=ControlSampleTime  ICPrevOutput=DiscIntNeverNeededParam  ICPrevScaledInput=DiscIntNeverNeededParam
  Sum1 : Sum  Inputs=|+-
  E_fil : Outport  VectorParamsAs1DForOutWhenUnconnected=off
  wires:
  Sum1/1 -> Divide2/1
  Integrator/1 -> E_fil/1, Sum1/2  "E [pu]"
  Tau/1 -> Divide2/2
  E/1 -> Sum1/1
  Divide2/1 -> Integrator/1
  E0/1 -> Integrator/2

== system AC_base_1_VSM_2_22a/Variant Subsystem1/VSM/VSM1/VSM/CONTROL/VSMOC1/VSMOC/Subsystem ==
  first_run : Inport
  u_dq : Inport  Port=2
  u_dq_pll : Inport  Port=3
  phi_pll : Inport  Port=4
  Enable : EnablePort
  Complex to Magnitude-Angle : ComplexToMagnitudeAngle
  Demux : Demux  Outputs=2
  Real-Imag to Complex : RealImagToComplex
  Switch : Switch  Criteria=u2 > Threshold  SaturateOnIntegerOverflow=off  InputSameDT=off
  Switch1 : Switch  Criteria=u2 ~= 0  SaturateOnIntegerOverflow=off  InputSameDT=off
  "first_run " : InportShadow
  u_abs : Outport  InitialOutput=1  VectorParamsAs1DForOutWhenUnconnected=off
  u_ang : Outport  Port=2  InitialOutput=0  VectorParamsAs1DForOutWhenUnconnected=off
  wires:
  Complex to Magnitude-Angle/2 -> Switch/3
  "first_run "/1 -> Switch/2
  u_dq_pll/1 -> Switch1/1
  u_dq/1 -> Switch1/3
  first_run/1 -> Switch1/2
  Switch1/1 -> Demux/1
  Complex to Magnitude-Angle/1 -> u_abs/1
  Demux/2 -> Real-Imag to Complex/2
  Demux/1 -> Real-Imag to Complex/1
  Real-Imag to Complex/1 -> Complex to Magnitude-Angle/1
  phi_pll/1 -> Switch/1
  Switch/1 -> u_ang/1

== system AC_base_1_VSM_2_22a/Variant Subsystem1/VSM/VSM1/VSM/MANAGEMENT/sp_VSM/RateLimit/ratelimitspPQ ==
  rateup : Inport
  x : Inport  Port=2
  ratedown : Inport  Port=3
  x0 : Inport  Port=4
  Delay : Delay  DelayLength=1  InitialConditionSource=Input port  SampleTime=Ts
      settings: InputPortMap=u0,p4
  Gain : Gain  Gain=Ts
  Gain1 : Gain  Gain=-Ts
  Saturation Dynamic2 : simulink/Discontinuities/Saturation Dynamic  OutMin=[]  OutMax=[]  OutDataTypeStr=Inherit: Same as second input  OutDataType=fixdt(1, 16)  OutScaling=2^-10  DoSatur=off
  Sum : Sum  Inputs=|+-
  Sum1 : Sum  Inputs=|++
  x_slow : Outport  VectorParamsAs1DForOutWhenUnconnected=off
  wires:
  x/1 -> Sum/1
  Delay/1 -> Sum1/2, Sum/2
  Sum/1 -> Saturation Dynamic2/2
  Saturation Dynamic2/1 -> Sum1/1
  Sum1/1 -> x_slow/1, Delay/1
  x0/1 -> Delay/2
  Gain/1 -> Saturation Dynamic2/1
  rateup/1 -> Gain/1
  ratedown/1 -> Gain1/1
  Gain1/1 -> Saturation Dynamic2/3

== system AC_base_1_VSM_2_22a/Variant Subsystem3/VSM/VSM1/VSM/CONTROL/VSMOC1/VSMOC/Enabled Subsystem ==
  u_abs : Inport
  Enable : EnablePort
  Out1 : Outport
  wires:
  u_abs/1 -> Out1/1

== system AC_base_1_VSM_2_22a/Variant Subsystem3/VSM/VSM1/VSM/CONTROL/VSMOC1/VSMOC/Enabled Subsystem1 ==
  P : Inport
  Enable : EnablePort
  Out1 : Outport
  wires:
  P/1 -> Out1/1

== system AC_base_1_VSM_2_22a/Variant Subsystem3/VSM/VSM1/VSM/CONTROL/VSMOC1/VSMOC/FRT Slow Down ==
  U : Inport
  Bias : Bias  Bias=0.2  SaturateOnIntegerOverflow=off
  Complex to Magnitude-Angle : ComplexToMagnitudeAngle
  Demux : Demux  Outputs=2
  Real-Imag to Complex : RealImagToComplex
  Saturation : Saturate  UpperLimit=1  LowerLimit=0
  Terminator : Terminator
  Unit Delay4 : UnitDelay  SampleTime=ControlSampleTime  HasFrameUpgradeWarning=on
  K : Outport  VectorParamsAs1DForOutWhenUnconnected=off
  wires:
  Complex to Magnitude-Angle/1 -> Bias/1
  Demux/2 -> Real-Imag to Complex/2
  Demux/1 -> Real-Imag to Complex/1
  Real-Imag to Complex/1 -> Complex to Magnitude-Angle/1
  U/1 -> Unit Delay4/1
  Complex to Magnitude-Angle/2 -> Terminator/1
  Bias/1 -> Saturation/1
  Saturation/1 -> K/1
  Unit Delay4/1 -> Demux/1

== system AC_base_1_VSM_2_22a/Variant Subsystem3/VSM/VSM1/VSM/CONTROL/VSMOC1/VSMOC/Integrator (Angle) ==
  Reset : Inport
  omega : Inport  Port=2
  d_phi0 : Inport  Port=3
  Angle Integrator Reset[SI] : FriedrichLibrary/Discrete Stuff/Angle Integrator Reset[SI]  Ts=ControlSampleTime
  Delay : Delay  DelayLength=1  InitialConditionSource=Input port
      settings: InputPortMap=u0,p4
  Gain3 : Gain  Gain=-1*ControlSampleTime
  Scope : Scope  NumInputPorts=2
  Scope1 : Scope  NumInputPorts=2
  Sum1 : Sum  Inputs=|++
  Sum9 : Sum  Inputs=|+-
  phi : Outport  VectorParamsAs1DForOutWhenUnconnected=off
  wires:
  Gain3/1 -> Sum9/2, Scope/2, Delay/2
  omega/1 -> Gain3/1, Angle Integrator Reset[SI]/2
  Angle Integrator Reset[SI]/1 -> Delay/1, phi/1  "Phi [rad]"
  Reset/1 -> Scope1/1, Angle Integrator Reset[SI]/1
  Sum9/1 -> Sum1/1
  Sum1/1 -> Scope1/2, Angle Integrator Reset[SI]/3
  d_phi0/1 -> Sum9/1
  Delay/1 -> Scope/1, Sum1/2

== system AC_base_1_VSM_2_22a/Variant Subsystem3/VSM/VSM1/VSM/CONTROL/VSMOC1/VSMOC/Integrator (Inertia) ==
  dPTa : Inport
  omega0 [pu] : Inport  Port=2
  Enable : EnablePort
  Integrator (inertia) : DiscreteIntegrator  gainval=1  InitialConditionSource=external  InitialCondition=1  SampleTime=ControlSampleTime  ICPrevOutput=DiscIntNeverNeededParam  ICPrevScaledInput=DiscIntNeverNeededParam
  omega [pu] : Outport  VectorParamsAs1DForOutWhenUnconnected=off
  wires:
  omega0 [pu]/1 -> Integrator (inertia)/2
  Integrator (inertia)/1 -> omega [pu]/1  "Omega [pu]"
  dPTa/1 -> Integrator (inertia)/1

== system AC_base_1_VSM_2_22a/Variant Subsystem3/VSM/VSM1/VSM/CONTROL/VSMOC1/VSMOC/P Filter Init ==
  Tau : Inport
  dP0 : Inport  Port=2
  Enable : EnablePort  StatesWhenEnabling=reset
  Divide4 : Product  Inputs=*/
  Gain : Gain  Gain=-1
  Integrator1 : DiscreteIntegrator  gainval=1  InitialConditionSource=external  SampleTime=ControlSampleTime  ICPrevOutput=DiscIntNeverNeededParam  ICPrevScaledInput=DiscIntNeverNeededParam
  dP : Outport  VectorParamsAs1DForOutWhenUnconnected=off
  wires:
  dP0/1 -> Integrator1/2
  Gain/1 -> Divide4/1
  Divide4/1 -> Integrator1/1
  Tau/1 -> Divide4/2
  Integrator1/1 -> dP/1, Gain/1

== system AC_base_1_VSM_2_22a/Variant Subsystem3/VSM/VSM1/VSM/CONTROL/VSMOC1/VSMOC/Q(U)-PI-Regler ==
  Tau : Inport
  E : Inport  Port=2
  E0 : Inport  Port=3
  Enable : EnablePort  StatesWhenEnabling=reset
  Divide2 : Product  Inputs=*/
  Integrator : DiscreteIntegrator  gainval=1  InitialConditionSource=external  InitialCondition=0.9  SampleTime=ControlSampleTime  ICPrevOutput=DiscIntNeverNeededParam  ICPrevScaledInput=DiscIntNeverNeededParam
  Sum1 : Sum  Inputs=|+-
  E_fil : Outport  VectorParamsAs1DForOutWhenUnconnected=off
  wires:
  E0/1 -> Integrator/2
  Divide2/1 -> Integrator/1
  E/1 -> Sum1/1
  Tau/1 -> Divide2/2
  Integrator/1 -> Sum1/2, E_fil/1  "E [pu]"
  Sum1/1 -> Divide2/1

== system AC_base_1_VSM_2_22a/Variant Subsystem3/VSM/VSM1/VSM/CONTROL/VSMOC1/VSMOC/Subsystem ==
  first_run : Inport
  u_dq : Inport  Port=2
  u_dq_pll : Inport  Port=3
  phi_pll : Inport  Port=4
  Enable : EnablePort
  Complex to Magnitude-Angle : ComplexToMagnitudeAngle
  Demux : Demux  Outputs=2
  Real-Imag to Complex : RealImagToComplex
  Switch : Switch  Criteria=u2 > Threshold  SaturateOnIntegerOverflow=off  InputSameDT=off
  Switch1 : Switch  Criteria=u2 ~= 0  SaturateOnIntegerOverflow=off  InputSameDT=off
  "first_run " : InportShadow
  u_abs : Outport  InitialOutput=1  VectorParamsAs1DForOutWhenUnconnected=off
  u_ang : Outport  Port=2  InitialOutput=0  VectorParamsAs1DForOutWhenUnconnected=off
  wires:
  Switch/1 -> u_ang/1
  phi_pll/1 -> Switch/1
  Real-Imag to Complex/1 -> Complex to Magnitude-Angle/1
  Demux/1 -> Real-Imag to Complex/1
  Demux/2 -> Real-Imag to Complex/2
  Complex to Magnitude-Angle/1 -> u_abs/1
  Switch1/1 -> Demux/1
  first_run/1 -> Switch1/2
  u_dq/1 -> Switch1/3
  u_dq_pll/1 -> Switch1/1
  "first_run "/1 -> Switch/2
  Complex to Magnitude-Angle/2 -> Switch/3

== system AC_base_1_VSM_2_22a/Variant Subsystem3/VSM/VSM1/VSM/MANAGEMENT/sp_VSM/RateLimit/ratelimitspPQ ==
  rateup : Inport
  x : Inport  Port=2
  ratedown : Inport  Port=3
  x0 : Inport  Port=4
  Delay : Delay  DelayLength=1  InitialConditionSource=Input port  SampleTime=Ts
      settings: InputPortMap=u0,p4
  Gain : Gain  Gain=Ts
  Gain1 : Gain  Gain=-Ts
  Saturation Dynamic2 : simulink/Discontinuities/Saturation Dynamic  OutMin=[]  OutMax=[]  OutDataTypeStr=Inherit: Same as second input  OutDataType=fixdt(1, 16)  OutScaling=2^-10  DoSatur=off
  Sum : Sum  Inputs=|+-
  Sum1 : Sum  Inputs=|++
  x_slow : Outport  VectorParamsAs1DForOutWhenUnconnected=off
  wires:
  Gain1/1 -> Saturation Dynamic2/3
  ratedown/1 -> Gain1/1
  rateup/1 -> Gain/1
  Gain/1 -> Saturation Dynamic2/1
  x0/1 -> Delay/2
  Sum1/1 -> Delay/1, x_slow/1
  Saturation Dynamic2/1 -> Sum1/1
  Sum/1 -> Saturation Dynamic2/2
  Delay/1 -> Sum/2, Sum1/2
  x/1 -> Sum/1

== matlab function AC_base_1_VSM_2_22a/Variant Subsystem1/VSM/VSM1/VSM/MANAGEMENT/Subsystem1/Subsystem/MATLAB Function2 ==
  data: i_inv input; i_sp output; PQ_out input; CC output; i_abs input; der input; set1 output; U_cap input; U_der1 input; U_der2 input
function [i_sp, CC, set1]= fcn(i_inv, PQ_out, i_abs, der, U_cap, U_der1, U_der2)
    persistent set
    if isempty(set)
        set = 0;
    end

    persistent d
    if isempty(d)
        d = 0;
    end    
    
    persistent x
    if isempty(x)
        x = 0;
    end    
    
    persistent i_sp_old
    if isempty(i_sp_old)
        i_sp_old = [0 0];
    end
    
    persistent a
    if isempty(a)
        a = [10 10 10 10];
    end
    
    persistent a_u
    if isempty(a_u)
        a_u = [10 10 10 10];
    end
    
    persistent zero
    if isempty(zero)
        zero = [10 10 10 10];
    end  
    
    persistent time
      if isempty(time)
        time = 0;
      end    
    time = time +1;
    
    persistent regler
    if isempty(regler)
        regler = 0;
    end    
    persistent sdf
    if isempty(sdf)
        sdf = 1;
    end  

    CC = false;
    i_sp = [0 0];
    f = 0;
    adf = 10;
    %i_abs = sqrt(i_inv(1)^2 + i_inv(2)^2 + i_inv(3)^2);
    
    if i_abs >= 1.2 && d == 0 % && U_cap <= 0.9 %momentan hohe Spannung
        CC = true;
        set = 1;
    end
    
    if set == 1
        
      i_sp = [0 0];
   CC = true;
    end
    
    if i_abs <= 1 && set == 1 %&& sum(a>1) <= 1
        
        set = 2;
        
        i_sp_old = [i_inv(1) i_inv(2)];
       CC = true;

    end
    a = [a(2:4) i_abs];
    a_u = [a_u(2:4) PQ_out(2)/U_cap];
    
    if set == 2 %&& sum(a>1) <= 1 %&& sum(a_u>0.4) == 0
        [angle, mag] = cart2pol(i_sp_old(1), i_sp_old(2));
        d = 2;
        if PQ_out(2)/U_cap <=0
            f = 6;
        else
        f = 6*(1 - PQ_out(2)/U_cap);            %%lieber PI benutzen und/oder Faktoren in Abhängigkeit von dU machen
        %f = ( PQ_out(2)/U_cap/0.5)^0.5;
        end
        regler = regler - 0.1*(1 - PQ_out(2)/U_cap)+angle*sdf;
i_sp = [regler, 1];
sdf=0;
     %   regler = regler + 0.98 - PQ_out(2)/U_cap;
%f = regler*0.1;
%         if abs(0-U_der1)<= 0.5
%             zero = [zero(2:4) 0]
%         else
%             zero = [zero(2:4) 10]
%         end
%         
%         if sum(zero) == 0 && U_der2 <0
%             f = 0;
%         end
        
        %i_sp = [angle-1/100*f, 1];
        
        [i_sp(1), i_sp(2)]  = pol2cart(i_sp(1), i_sp(2));
        
%         if sum(zero) == 0 && U_der2 <0
%             set = 3;
%             i_sp = [i_inv(1) i_inv(2)];
%         end
        i_sp_old = i_sp;
        CC = true;
        
%         if U_der2 <= 0 && abs(0-U_der1)<= 0.5
%             
%             f = 0;
%         end
%         


    end
    
%     letzte Bedingung ist ungünstig. Entweder Erfüllung des
%     Stromsollwertes mit i_sp~=0, oder Counter in set 2
    
%     if abs(PQ_out(1)) <= 0.05 && PQ_out(2) > 0 && set == 2 && sqrt(PQ_out(1)^2 + PQ_out(2)^2) > 0.1
%               
%        set = 3
%        
%        %i_sp_old = [i_inv(1) i_inv(2)];          % nimmt den aktuellen Stromwert für Blindstrombestimmung
%         CC = true;
%     end    

    if PQ_out(2)/U_cap >= 0.98 && set == 2 %&& sum(a_u>0.4) == 4 
        %set = 3;
        CC = true;
        adf = 20;
              %  CC = false;
        %set = 0;
       % i_sp_old = [0 0];
    end

    if set == 3
       
     % i_sp = i_sp_old * (1 - U_cap);
      i_sp = i_sp_old * 1;
      %i_sp = [0.28 -1.06];
       CC = true;
x = x +1;

    if x >= 50
        set = 4;
        CC = false;
        x = 0;
        i_sp_old = [0 0];
    end
    end
    
   if 0.115 == time/8000 
        set = 4;
        CC = false;
        x = 0;
        i_sp_old = [0 0];
    end
%     
%     % Regelabweichung nicht sonderlich relevant-> lässt CC nur länger
%     % ausgelöst
%     
%     if set == 3 && abs(der(1)) <= 5 && abs(der(2)) <= 5 && abs(i_inv(1)-i_sp(1)) <= 0.05 && abs(i_inv(2)-i_sp(2)) <= 0.05
%         CC = false;
%         set = 0;
%         i_sp_old = [0 0];
%     end
%     

   
    
    %% Spannungswiederkehr ohne Überstrom
    
%     if U_cap >= 0.9
%         CC = true;
%         set = 5;
%         x= x +1;
%     end
%     
%     if x >= 2
%         CC = false;
%         set = 0;
%         x = 0;
%     end
%     %% Spannungswiederkehr
%     
    if i_abs >= 1.2 && U_cap >= 0.6 && set == 4
        CC = true;
        set = 5;
    end
    
    if set == 5
        
      i_sp = [0 0];
   CC = true;
    end
    
    if i_abs <= 0.8 && set == 5
        
        set = 6;
        
        i_sp_old = [i_inv(1) i_inv(2)];
       CC = true;

    end
    q=0;
    if set == 6
        [angle, mag] = cart2pol(i_sp_old(1), i_sp_old(2));
        
        %if PQ_out(1) <= 0.5
        f = 6*(0.83 - PQ_out(1));            %%lieber PI benutzen und/oder Faktoren in Abhängigkeit von dU machen
        %f = ( PQ_out(2)/U_cap/0.5)^0.5;
        %end
        q = 3*(0.28 - PQ_out(2));
        i_sp = [angle-1/100*f-1/100*q, 0.8];
        
        [i_sp(1), i_sp(2)]  = pol2cart(i_sp(1), i_sp(2));
        
        i_sp_old = i_sp;
        CC = true;     
    end
    
    if time/8000 >= 0.23
                CC = false;
        set = 0;
        i_sp_old = [0 0];
    end
        
% %     letzte Bedingung ist ungünstig. Entweder Erfüllung des
% %     Stromsollwertes mit i_sp~=0, oder Counter in set 2
%     
%     if abs(PQ_out(2)) <= 0.05 && PQ_out(1) > 0 && set == 6 && sqrt(PQ_out(1)^2 + PQ_out(2)^2) > 0.1
%               
%        set = 7
%         CC = true;
%     end    
%    
%     if set == 7
%        
%       i_sp = i_sp_old;
%        CC = true;
%     end
%     
%     % Regelabweichung nicht sonderlich relevant-> lässt CC nur länger
%     % ausgelöst
%     
%     if set == 7 && abs(der(1)) <= 10 && abs(der(2)) <= 10 && abs(i_inv(1)-i_sp(1)) <= 0.05 && abs(i_inv(2)-i_sp(2)) <= 0.05
%         CC = false;
%         set = 0;
%         i_sp_old = [0 0];
%     end
    [angle, mag] = cart2pol(i_sp_old(1), i_sp_old(2));
     set1 = set;%regler; %angle;

== matlab function AC_base_1_VSM_2_22a/Variant Subsystem1/VSM/VSM1/VSM/MANAGEMENT/current_watchdog/MATLAB Function ==
  data: abs input; CC output; set input; i output; p input; i_inv input
function [CC, i] = fcn(abs, set, p, i_inv)
CC = false;
i=[0 0]

if abs >= set
    CC = true;
    i=[1 1]
%     if PQ(1)<0.5
%         i=[0 1]
%     end
end

== matlab function AC_base_1_VSM_2_22a/Variant Subsystem3/VSM/VSM1/VSM/CONTROL/Subsystem1/MATLAB Function ==
  data: phi_vsm output; I input; L1 input; R1 input; U_i input; U_v output
function [phi_vsm, U_v]  = fcn(I, L1, R1, U_i)

% phi_vsm = 0;
% U_v = [0 ;0];
% I = [I(1); I(2)];
% Z = [R1 -L1; L1 R1];
% for n = -0.8-1:0.0005:2+1
%     phi = n;
% rot = [cos(phi) sin(phi); -sin(phi) cos(phi)];
% U_v = rot.'*([U_i(1); U_i(2)]+Z*I);
% if abs(0-U_v(2,1))<= 0.0005
%     phi_vsm = phi;
%     U_v;
%     break
% end
% end
    persistent phi
    if isempty(phi)
       phi = 0;
    end    
    
phi_vsm = 0;
U_v = [0 ;0];
I = [I(1); I(2)];
Z = [R1 -L1; L1 R1];

rot = [cos(phi) sin(phi); -sin(phi) cos(phi)];
U_v = rot.'*([U_i(1); U_i(2)]+Z*I);

diff = 0-U_v(2,1);
if abs(diff) >= 1
    diff =1;
end

phi = phi + 1*(diff);
phi_vsm = phi;
% if abs(0-U_v(2,1))<= 0.0005 geht so nicht, da nur eine Richtung
%     phi_vsm = phi;
%     U_v;
% else
%     phi = phi + 0.0005;
% end
